simulink model "PROYECTO_SIMULINK"  (R2023a)
settings: Solver=VariableStepAuto  StartTime=0.0  StopTime=10  MaxStep=1e-3  RelTol=1e-3
libraries: slpidlib x1
settings Model: Creator=abrah  LastModifiedBy=hp
settings DataIOCC: ReturnWorkspaceOutputs=off  TimeSaveName=t
settings DebuggingCC: AlgebraicLoopMsg=none

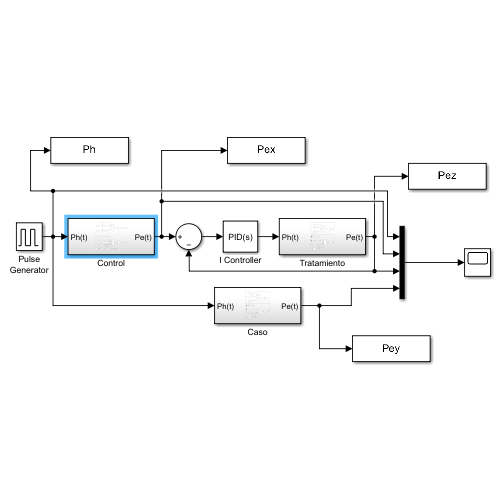
[thumbnail: Simulink's stored preview of the top-level diagram]
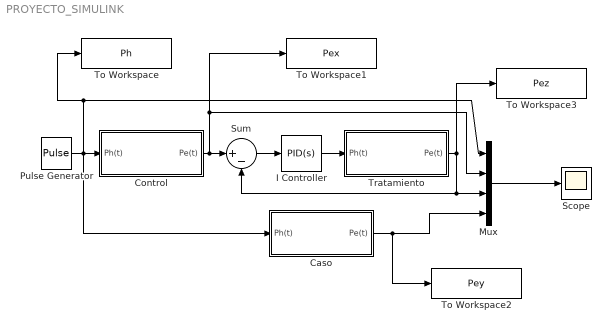
== system PROYECTO_SIMULINK ==
  Caso : Subsystem
  Control : Subsystem
  I Controller : slpidlib/PID Controller  Controller=PID  Form=Parallel  TimeDomain=Continuous-time  UseExternalTs=off  SampleTime=-1  IntegratorMethod=Forward Euler  FilterMethod=Forward Euler  ControllerParametersSource=internal  P=0  I=1317.4583  UseKiTs=off  D=0  N=100  UseFilter=on  TunerSelectOption=Transfer Function Based (PID Tuner App)  InitialConditionSource=internal  InitialConditionForIntegrator=0  InitialConditionForFilter=0  DifferentiatorICPrevScaledInput=0  ExternalReset=none  TrackingMode=off  Kt=1  LimitOutput=off  SatLimitsSource=internal  UpperSaturationLimit=inf  LowerSaturationLimit=-inf  LinearizeAsGain=on  AntiWindupMode=none  Kb=1  LimitIntegrator=off  UpperIntegratorSaturationLimit=inf  LowerIntegratorSaturationLimit=-inf  POutMin=[]  POutMax=[]  IOutMin=[]  IOutMax=[]  DOutMin=[]  DOutMax=[]  NOutMin=[]  NOutMax=[]  SumOutMin=[]  SumOutMax=[]  SaturationOutMin=[]  SaturationOutMax=[]  PParamMin=[]  PParamMax=[]  IParamMin=[]  IParamMax=[]  DParamMin=[]  DParamMax=[]  NParamMin=[]  NParamMax=[]  KbParamMin=[]  KbParamMax=[]  KtParamMin=[]  KtParamMax=[]  KbOutMin=[]  KbOutMax=[]  KtOutMin=[]  KtOutMax=[]  IntegratorOutMin=[]  IntegratorOutMax=[]  FilterOutMin=[]  FilterOutMax=[]  SumI1OutMin=[]  SumI1OutMax=[]  SumI2OutMin=[]  SumI2OutMax=[]  SumI3OutMin=[]  SumI3OutMax=[]  SumI4OutMin=[]  SumI4OutMax=[]  SumDOutMin=[]  SumDOutMax=[]  DifferentiatorOutMin=[]  DifferentiatorOutMax=[]  FilterDiffOutCoefMin=[]  FilterDiffOutCoefMax=[]  ReciprocalOutMin=[]  ReciprocalOutMax=[]  SumDenOutMin=[]  SumDenOutMax=[]  SumNumOutMin=[]  SumNumOutMax=[]  DivideOutMin=[]  DivideOutMax=[]  UdiffTsProdOutMin=[]  UdiffTsProdOutMax=[]  NTsProdOutMin=[]  NTsProdOutMax=[]  UintegralTsProdOutMin=[]  UintegralTsProdOutMax=[]  UngainTsProdOutMin=[]  UngainTsProdOutMax=[]  ClampingZeroOutDataTypeStr=Inherit: Inherit via back propagation  ClampingZeroOutMin=[]  ClampingZeroOutMax=[]  FilterDenConstantOutDataTypeStr=Inherit: Inherit via back propagation  FilterDenConstantOutMin=[]  FilterDenConstantOutMax=[]  PCopyOutDataTypeStr=Inherit: Inherit via back propagation  PCopyOutMin=[]  PCopyOutMax=[]  NCopyOutDataTypeStr=Inherit: Inherit via back propagation  NCopyOutMin=[]  NCopyOutMax=[]  IntegratorContinuousStateAttributes=''  IntegratorStateMustResolveToSignalObject=off  IntegratorRTWStateStorageClass=Auto  FilterContinuousStateAttributes=''  FilterStateMustResolveToSignalObject=off  FilterRTWStateStorageClass=Auto  ParallelPVariant=InternalParameters  IdealPVariant=Disabled  IVariant=InternalParameters  DVariant=InternalParameters  IntegratorVariant=Continuous  SatVariant=Disabled  AWVariant=Passthrough  PCopyVariant=Disabled  TRVariant=Disabled  FdbkBlocksVariant=Forward  IdealPFdbkVariant=Disabled  SatFdbkVariant=Disabled  DerivativeFilterVariant=ContFilter  NVariant=InternalParameters  NCopyVariant=Disabled  FilterICVariant=InternalICsFilter  IntegratorICVariant=InternalICs  ExternalResetVariant=Disabled  TRSumVariant=Passthrough  SumFdbkVariant=Disabled  SumVariant=Sum_PID  TsampFilterVariant=InternalTs  TsampNgainVariant=Passthrough  TsampIntegralVariant=Disabled_SignalSpec  ExternalSaturationOutDataTypeStr=Inherit: Same as second input
  Mux : Mux
  Pulse Generator : DiscretePulseGenerator  PulseType=Time based  Period=10  PulseWidth=10  PhaseDelay=1
  Scope : Scope
  Sum : Sum  Inputs=|+-
  To Workspace : ToWorkspace  VariableName=Ph  SampleTime=-1
  To Workspace1 : ToWorkspace  VariableName=Pex  SampleTime=-1
  To Workspace2 : ToWorkspace  VariableName=Pey  SampleTime=-1
  To Workspace3 : ToWorkspace  VariableName=Pez  SampleTime=-1
  Tratamiento : Subsystem
  wires:
  Mux/1 -> Scope/1
  Pulse Generator/1 -> To Workspace/1, Mux/1, Caso/1(Ph(t)), Control/1(Ph(t))
  Sum/1 -> I Controller/1
  Control/1(Pe(t)) -> To Workspace1/1, Mux/2, Sum/1
  I Controller/1 -> Tratamiento/1(Ph(t))
  Tratamiento/1(Pe(t)) -> To Workspace3/1, Sum/2, Mux/3
  Caso/1(Pe(t)) -> To Workspace2/1, Mux/4

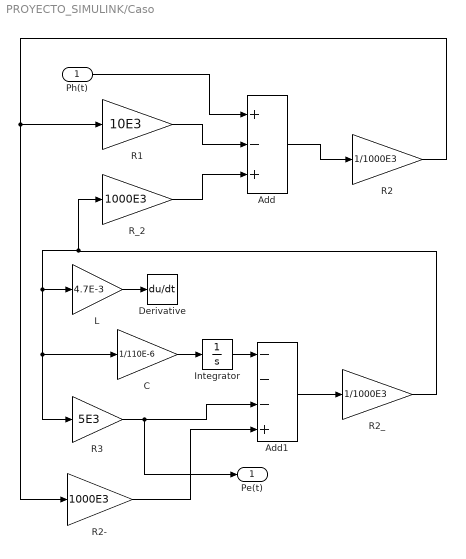
== system PROYECTO_SIMULINK/Caso ==
  Ph(t) : Inport
  Add : Sum  Inputs=+-+
  Add1 : Sum  Inputs=---+
  C : Gain  Gain=1/110E-6
  Derivative : Derivative
  Integrator : Integrator
  L : Gain  Gain=4.7E-3
  R1 : Gain  Gain=10E3
  R2 : Gain  Gain=1/1000E3
  R2- : Gain  Gain=1000E3
  R2_ : Gain  Gain=1/1000E3
  R3 : Gain  Gain=5E3
  R_2 : Gain  Gain=1000E3
  Pe(t) : Outport
  wires:
  Add/1 -> R2/1
  R1/1 -> Add/2
  R_2/1 -> Add/3
  R2_/1 -> R3/1, C/1, L/1, R_2/1
  Add1/1 -> R2_/1
  R3/1 -> Pe(t)/1, Add1/3
  R2-/1 -> Add1/4
  R2/1 -> R2-/1, R1/1
  Ph(t)/1 -> Add/1
  L/1 -> Derivative/1
  C/1 -> Integrator/1
  Integrator/1 -> Add1/1

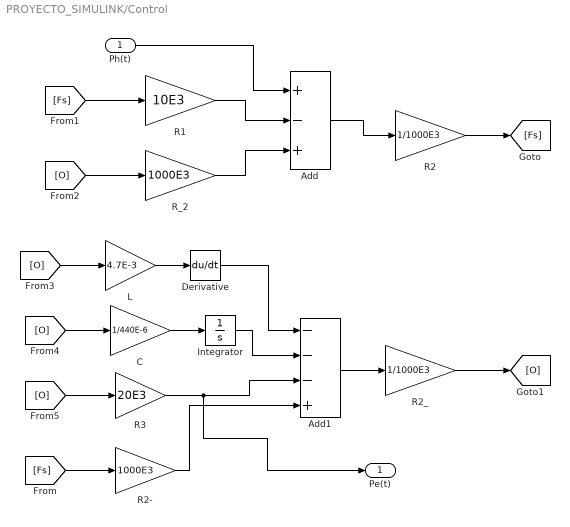
== system PROYECTO_SIMULINK/Control ==
  Ph(t) : Inport
  Add : Sum  Inputs=+-+
  Add1 : Sum  Inputs=---+
  C : Gain  Gain=1/440E-6
  Derivative : Derivative
  Integrator : Integrator
  L : Gain  Gain=4.7E-3
  R1 : Gain  Gain=10E3
  R2 : Gain  Gain=1/1000E3
  R2- : Gain  Gain=1000E3
  R2_ : Gain  Gain=1/1000E3
  R3 : Gain  Gain=20E3
  R_2 : Gain  Gain=1000E3
  Pe(t) : Outport
  wires:
  Ph(t)/1 -> Add/1
  Add/1 -> R2/1
  R2/1 -> [Fs]
  R1/1 -> Add/2
  [Fs] -> R1/1
  R_2/1 -> Add/3
  [O] -> R_2/1
  Add1/1 -> R2_/1
  R2_/1 -> [O]
  R3/1 -> Pe(t)/1, Add1/3
  [O] -> R3/1
  R2-/1 -> Add1/4
  [Fs] -> R2-/1
  L/1 -> Derivative/1
  C/1 -> Integrator/1
  Derivative/1 -> Add1/1
  Integrator/1 -> Add1/2
  [O] -> L/1
  [O] -> C/1

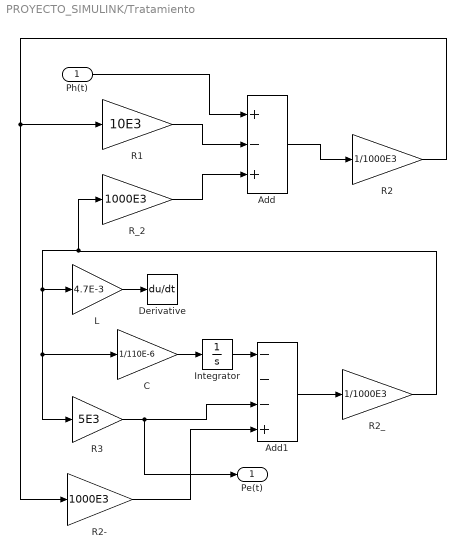
== system PROYECTO_SIMULINK/Tratamiento ==
  Ph(t) : Inport
  Add : Sum  Inputs=+-+
  Add1 : Sum  Inputs=---+
  C : Gain  Gain=1/110E-6
  Derivative : Derivative
  Integrator : Integrator
  L : Gain  Gain=4.7E-3
  R1 : Gain  Gain=10E3
  R2 : Gain  Gain=1/1000E3
  R2- : Gain  Gain=1000E3
  R2_ : Gain  Gain=1/1000E3
  R3 : Gain  Gain=5E3
  R_2 : Gain  Gain=1000E3
  Pe(t) : Outport
  wires:
  Integrator/1 -> Add1/1
  C/1 -> Integrator/1
  R2-/1 -> Add1/4
  R2/1 -> R2-/1, R1/1
  L/1 -> Derivative/1
  Ph(t)/1 -> Add/1
  Add1/1 -> R2_/1
  R3/1 -> Pe(t)/1, Add1/3
  Add/1 -> R2/1
  R_2/1 -> Add/3
  R1/1 -> Add/2
  R2_/1 -> R3/1, C/1, L/1, R_2/1
